simulink model "counter_cascaded"  (R2014a)
settings: Solver=FixedStepDiscrete  StartTime=0.0  StopTime=1000  FixedStep=1  RelTol=1e-3
libraries: hdlsllib x2, simulink x1
settings Model: Creator=Andrew  LastModifiedBy=Andrew

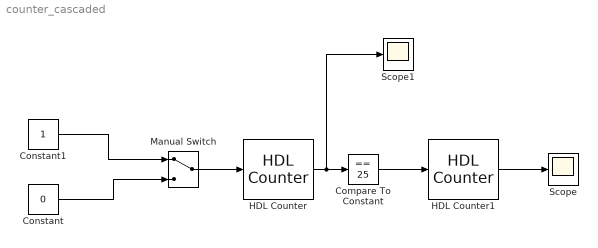
== system counter_cascaded ==
  Compare To Constant : simulink/Logic and Bit Operations/Compare To Constant  relop===  const=25  OutDataTypeStr=boolean
  Constant : Constant  Value=0  OutDataTypeStr=boolean
  Constant1 : Constant  OutDataTypeStr=boolean
  HDL Counter : hdlsllib/HDL Operations/HDL Counter  CountType=Free running  CountInit=0  CountStep=1  CountMax=100  CountFromType=Initial value  CountFrom=0  CountResetPort=off  CountLoadPort=off  CountEnbPort=on  CountDirPort=off  CountDataType=Unsigned  CountWordLen=8  CountFracLen=0  CountSampTime=1
  HDL Counter1 : hdlsllib/HDL Operations/HDL Counter  CountType=Free running  CountInit=0  CountStep=1  CountMax=100  CountFromType=Initial value  CountFrom=0  CountResetPort=off  CountLoadPort=off  CountEnbPort=on  CountDirPort=off  CountDataType=Unsigned  CountWordLen=8  CountFracLen=0  CountSampTime=1
  Manual Switch : ManualSwitch
  Scope : Scope
  Scope1 : Scope
  wires:
  Constant1/1 -> Manual Switch/1
  Constant/1 -> Manual Switch/2
  Manual Switch/1 -> HDL Counter/1
  HDL Counter/1 -> Scope1/1, Compare To Constant/1
  Compare To Constant/1 -> HDL Counter1/1
  HDL Counter1/1 -> Scope/1
